simulink model "gm_Prediction_and_cost_function_FCS_MPC_6Phase_PMSM"  (R2022a)
settings: Solver=FixedStepDiscrete  StartTime=0.0  StopTime=10.0  RelTol=1e-3
undefined symbols (not defined in the file or in its folder): f_c, L_d, L_q, L_x, L_y, p, psi_pm, R_ph
libraries: hdlmdlgenlib x6
(part 2 of 2)

== system gm_Prediction_and_cost_function_FCS_MPC_6Phase_PMSM/HDL_DUT/MATLAB Function/square3 ==
  In1 : Inport
  In2 : Inport  Port=2
  square3 : Product  Inputs=**  OutDataTypeStr=single  SampleTime=1e-08
  square3_pd1 : Delay  DelayLength=8
  Out1 : Outport
  wires:
  In1/1 -> square3/1
  In2/1 -> square3/2
  square3/1 -> square3_pd1/1
  square3_pd1/1 -> Out1/1

== system gm_Prediction_and_cost_function_FCS_MPC_6Phase_PMSM/HDL_DUT/MATLAB Function/subtract ==
  In1 : Inport
  In2 : Inport  Port=2
  subtract : Sum  Inputs=+-  OutDataTypeStr=single  SampleTime=1e-08
  subtract_pd1 : Delay  DelayLength=11
  Out1 : Outport
  wires:
  In1/1 -> subtract/1
  In2/1 -> subtract/2
  subtract/1 -> subtract_pd1/1
  subtract_pd1/1 -> Out1/1

== system gm_Prediction_and_cost_function_FCS_MPC_6Phase_PMSM/HDL_DUT/MATLAB Function/subtract1 ==
  In1 : Inport
  In2 : Inport  Port=2
  subtract1 : Sum  Inputs=+-  OutDataTypeStr=single  SampleTime=1e-08
  subtract1_pd1 : Delay  DelayLength=11
  Out1 : Outport
  wires:
  In1/1 -> subtract1/1
  In2/1 -> subtract1/2
  subtract1/1 -> subtract1_pd1/1
  subtract1_pd1/1 -> Out1/1

== system gm_Prediction_and_cost_function_FCS_MPC_6Phase_PMSM/HDL_DUT/MATLAB Function/subtract2 ==
  In1 : Inport
  In2 : Inport  Port=2
  subtract2 : Sum  Inputs=+-  OutDataTypeStr=single  SampleTime=1e-08
  subtract2_pd1 : Delay  DelayLength=11
  Out1 : Outport
  wires:
  In1/1 -> subtract2/1
  In2/1 -> subtract2/2
  subtract2/1 -> subtract2_pd1/1
  subtract2_pd1/1 -> Out1/1

== system gm_Prediction_and_cost_function_FCS_MPC_6Phase_PMSM/HDL_DUT/MATLAB Function/subtract3 ==
  In1 : Inport
  In2 : Inport  Port=2
  subtract3 : Sum  Inputs=+-  OutDataTypeStr=single  SampleTime=1e-08
  subtract3_pd1 : Delay  DelayLength=11
  Out1 : Outport
  wires:
  In1/1 -> subtract3/1
  In2/1 -> subtract3/2
  subtract3/1 -> subtract3_pd1/1
  subtract3_pd1/1 -> Out1/1

== system gm_Prediction_and_cost_function_FCS_MPC_6Phase_PMSM/HDL_DUT/MATLAB Function/subtract4 ==
  In1 : Inport
  In2 : Inport  Port=2
  subtract4 : Sum  Inputs=+-  OutDataTypeStr=single  SampleTime=1e-08
  subtract4_pd1 : Delay  DelayLength=11
  Out1 : Outport
  wires:
  In1/1 -> subtract4/1
  In2/1 -> subtract4/2
  subtract4/1 -> subtract4_pd1/1
  subtract4_pd1/1 -> Out1/1

== system gm_Prediction_and_cost_function_FCS_MPC_6Phase_PMSM/HDL_DUT/MATLAB Function/subtract5 ==
  In1 : Inport
  In2 : Inport  Port=2
  subtract5 : Sum  Inputs=+-  OutDataTypeStr=single  SampleTime=1e-08
  subtract5_pd1 : Delay  DelayLength=11
  Out1 : Outport
  wires:
  In1/1 -> subtract5/1
  In2/1 -> subtract5/2
  subtract5/1 -> subtract5_pd1/1
  subtract5_pd1/1 -> Out1/1

== system gm_Prediction_and_cost_function_FCS_MPC_6Phase_PMSM/HDL_DUT/MATLAB Function/subtract6 ==
  In1 : Inport
  In2 : Inport  Port=2
  subtract6 : Sum  Inputs=+-  OutDataTypeStr=single  SampleTime=1e-08
  subtract6_pd1 : Delay  DelayLength=11
  Out1 : Outport
  wires:
  In1/1 -> subtract6/1
  In2/1 -> subtract6/2
  subtract6/1 -> subtract6_pd1/1
  subtract6_pd1/1 -> Out1/1

== system gm_Prediction_and_cost_function_FCS_MPC_6Phase_PMSM/HDL_DUT/MATLAB Function/subtract7 ==
  In1 : Inport
  In2 : Inport  Port=2
  subtract7 : Sum  Inputs=+-  OutDataTypeStr=single  SampleTime=1e-08
  subtract7_pd1 : Delay  DelayLength=11
  Out1 : Outport
  wires:
  In1/1 -> subtract7/1
  In2/1 -> subtract7/2
  subtract7/1 -> subtract7_pd1/1
  subtract7_pd1/1 -> Out1/1

== system gm_Prediction_and_cost_function_FCS_MPC_6Phase_PMSM/HDL_DUT/MATLAB Function/subtract8 ==
  In1 : Inport
  In2 : Inport  Port=2
  subtract8 : Sum  Inputs=+-  OutDataTypeStr=single  SampleTime=1e-08
  subtract8_pd1 : Delay  DelayLength=11
  Out1 : Outport
  wires:
  In1/1 -> subtract8/1
  In2/1 -> subtract8/2
  subtract8/1 -> subtract8_pd1/1
  subtract8_pd1/1 -> Out1/1
